simulink library "ServoCommand"  (R2014b)
settings: Solver=ode45  StartTime=0.0  StopTime=10.0  RelTol=1e-3
libraries: ServoCommand x12, simulink x6
settings Model: Creator=Sebastian  LastModifiedBy=Sebastian

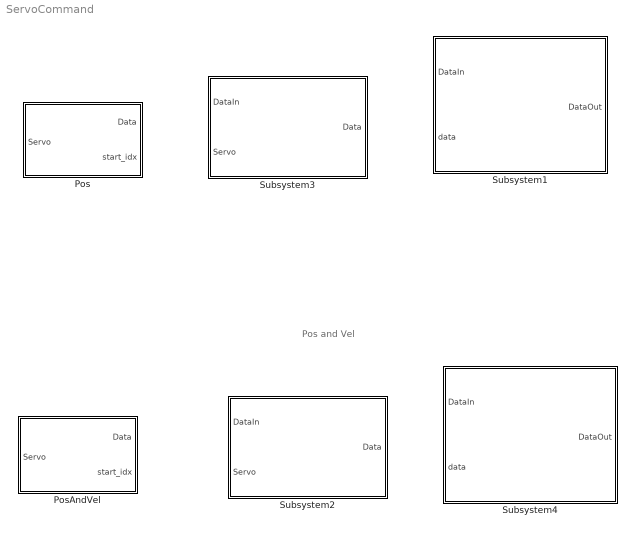
== system ServoCommand ==
  note: Pos and Vel
  Pos : Subsystem
  PosAndVel : Subsystem
  Subsystem1 : Subsystem
  Subsystem2 : Subsystem
  Subsystem3 : Subsystem
  Subsystem4 : Subsystem

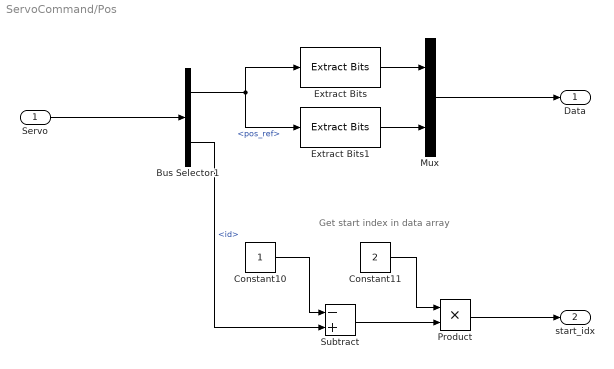
== system ServoCommand/Pos ==
  note: Get start index in data array
  Servo : Inport
  Bus Selector1 : BusSelector  OutputSignals=pos_ref,id
  Constant10 : Constant  OutDataTypeStr=uint8  SampleTime=-1
  Constant11 : Constant  Value=2  OutDataTypeStr=uint8  SampleTime=-1
  Extract Bits : simulink/Logic and Bit Operations/Extract Bits  bitsToExtract=Lower half  numBits=8  bitIdxRange=[0 7]  outScalingMode=Treat bit field as an integer
  Extract Bits1 : simulink/Logic and Bit Operations/Extract Bits  bitsToExtract=Upper half  numBits=8  bitIdxRange=[0 7]  outScalingMode=Treat bit field as an integer
  Mux : Mux  Inputs=2
  Product : Product
  Subtract : Sum  Inputs=-+
  Data : Outport
  start_idx : Outport  Port=2
  wires:
  Extract Bits/1 -> Mux/1
  Extract Bits1/1 -> Mux/2
  Servo/1 -> Bus Selector1/1
  Bus Selector1/1 -> Extract Bits/1, Extract Bits1/1  "<pos_ref>"
  Constant10/1 -> Subtract/1
  Subtract/1 -> Product/2
  Product/1 -> start_idx/1
  Constant11/1 -> Product/1
  Bus Selector1/2 -> Subtract/2  "<id>"
  Mux/1 -> Data/1

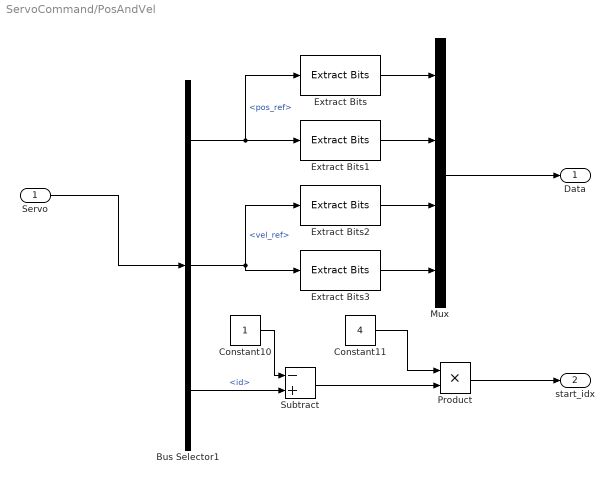
== system ServoCommand/PosAndVel ==
  Servo : Inport  OutDataTypeStr=Bus: Servo
  Bus Selector1 : BusSelector  OutputSignals=pos_ref,vel_ref,id
  Constant10 : Constant  OutDataTypeStr=uint8  SampleTime=-1
  Constant11 : Constant  Value=4  OutDataTypeStr=uint8  SampleTime=-1
  Extract Bits : simulink/Logic and Bit Operations/Extract Bits  bitsToExtract=Lower half  numBits=8  bitIdxRange=[0 7]  outScalingMode=Treat bit field as an integer
  Extract Bits1 : simulink/Logic and Bit Operations/Extract Bits  bitsToExtract=Upper half  numBits=8  bitIdxRange=[0 7]  outScalingMode=Treat bit field as an integer
  Extract Bits2 : simulink/Logic and Bit Operations/Extract Bits  bitsToExtract=Lower half  numBits=8  bitIdxRange=[0 7]  outScalingMode=Treat bit field as an integer
  Extract Bits3 : simulink/Logic and Bit Operations/Extract Bits  bitsToExtract=Upper half  numBits=8  bitIdxRange=[0 7]  outScalingMode=Treat bit field as an integer
  Mux : Mux
  Product : Product
  Subtract : Sum  Inputs=-+
  Data : Outport
  start_idx : Outport  Port=2
  wires:
  Extract Bits/1 -> Mux/1
  Extract Bits1/1 -> Mux/2
  Servo/1 -> Bus Selector1/1
  Bus Selector1/1 -> Extract Bits/1, Extract Bits1/1  "<pos_ref>"
  Constant10/1 -> Subtract/1
  Subtract/1 -> Product/2
  Product/1 -> start_idx/1
  Constant11/1 -> Product/1
  Bus Selector1/3 -> Subtract/2  "<id>"
  Mux/1 -> Data/1
  Extract Bits2/1 -> Mux/3
  Extract Bits3/1 -> Mux/4
  Bus Selector1/2 -> Extract Bits2/1, Extract Bits3/1  "<vel_ref>"

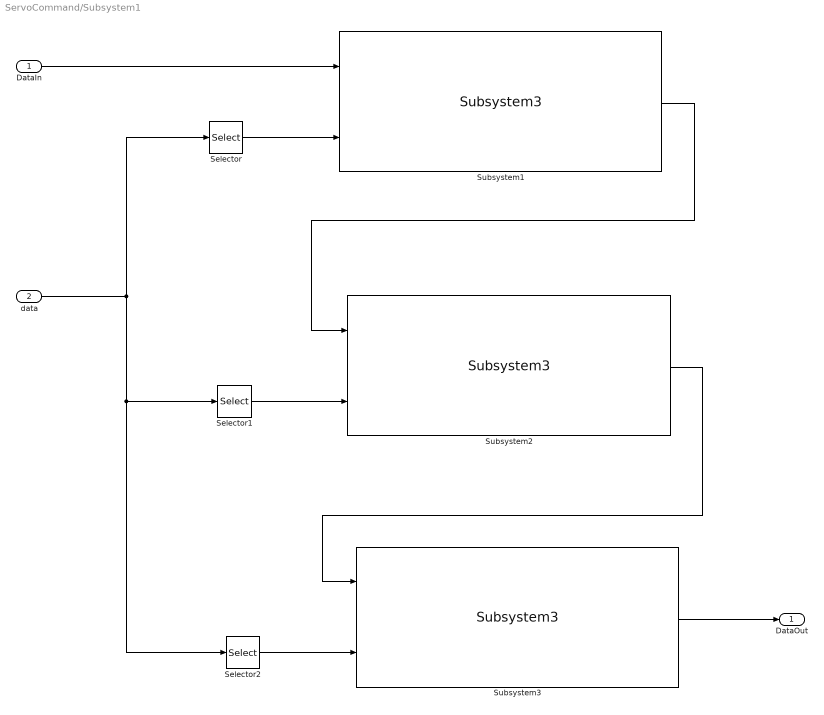
== system ServoCommand/Subsystem1 ==
  DataIn : Inport
  data : Inport  Port=2
  Selector : Selector  IndexMode=Zero-based  InputPortWidth=3  Indices=0
  Selector1 : Selector  IndexMode=Zero-based  InputPortWidth=3
  Selector2 : Selector  IndexMode=Zero-based  InputPortWidth=3  Indices=2
  Subsystem1 : ServoCommand/Subsystem3
  Subsystem2 : ServoCommand/Subsystem3
  Subsystem3 : ServoCommand/Subsystem3
  DataOut : Outport
  wires:
  Selector1/1 -> Subsystem2/2
  Subsystem2/1 -> Subsystem3/1
  data/1 -> Selector1/1, Selector2/1, Selector/1
  Selector2/1 -> Subsystem3/2
  Subsystem1/1 -> Subsystem2/1
  DataIn/1 -> Subsystem1/1
  Selector/1 -> Subsystem1/2
  Subsystem3/1 -> DataOut/1

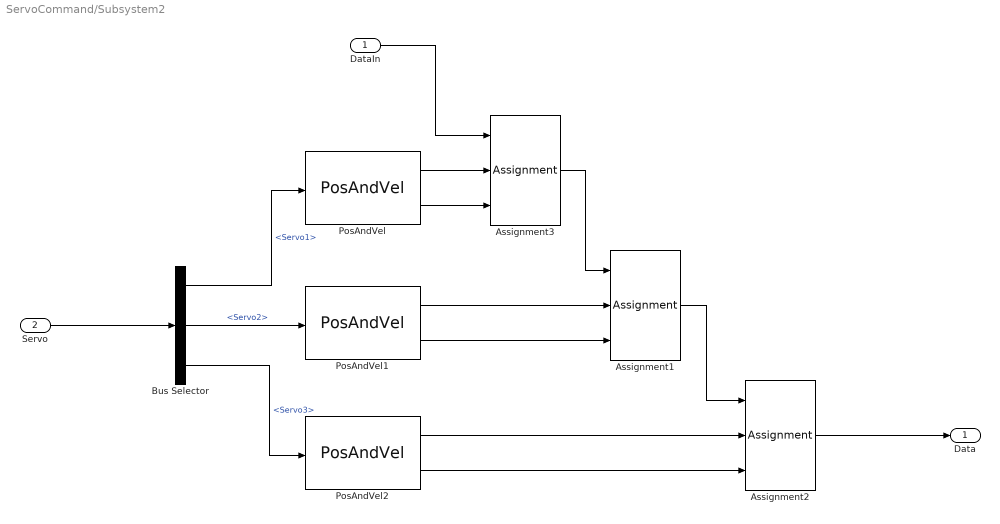
== system ServoCommand/Subsystem2 ==
  DataIn : Inport
  Servo : Inport  Port=2  OutDataTypeStr=Bus: Leg_ref
  Assignment1 : Assignment  IndexMode=Zero-based  IndexOptions=Starting index (port)  OutputSizes=36
  Assignment2 : Assignment  IndexMode=Zero-based  IndexOptions=Starting index (port)  OutputSizes=36
  Assignment3 : Assignment  IndexMode=Zero-based  IndexOptions=Starting index (port)  OutputSizes=36
  Bus Selector : BusSelector  OutputSignals=Servo1,Servo2,Servo3
  PosAndVel : ServoCommand/PosAndVel
  PosAndVel1 : ServoCommand/PosAndVel
  PosAndVel2 : ServoCommand/PosAndVel
  Data : Outport
  wires:
  Servo/1 -> Bus Selector/1
  Assignment2/1 -> Data/1
  DataIn/1 -> Assignment3/1
  PosAndVel2/2 -> Assignment2/3
  PosAndVel/1 -> Assignment3/2
  Bus Selector/3 -> PosAndVel2/1  "<Servo3>"
  PosAndVel/2 -> Assignment3/3
  PosAndVel1/1 -> Assignment1/2
  PosAndVel1/2 -> Assignment1/3
  Assignment1/1 -> Assignment2/1
  PosAndVel2/1 -> Assignment2/2
  Assignment3/1 -> Assignment1/1
  Bus Selector/2 -> PosAndVel1/1  "<Servo2>"
  Bus Selector/1 -> PosAndVel/1  "<Servo1>"

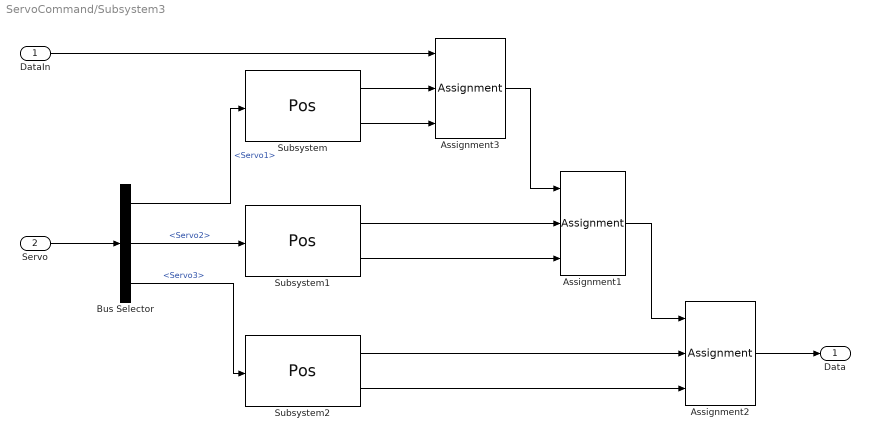
== system ServoCommand/Subsystem3 ==
  DataIn : Inport
  Servo : Inport  Port=2  OutDataTypeStr=Bus: Leg_ref
  Assignment1 : Assignment  IndexMode=Zero-based  IndexOptions=Starting index (port)  OutputSizes=36
  Assignment2 : Assignment  IndexMode=Zero-based  IndexOptions=Starting index (port)  OutputSizes=36
  Assignment3 : Assignment  IndexMode=Zero-based  IndexOptions=Starting index (port)  OutputSizes=36
  Bus Selector : BusSelector  OutputSignals=Servo1,Servo2,Servo3
  Subsystem : ServoCommand/Pos
  Subsystem1 : ServoCommand/Pos
  Subsystem2 : ServoCommand/Pos
  Data : Outport
  wires:
  Servo/1 -> Bus Selector/1
  Assignment2/1 -> Data/1
  Subsystem2/2 -> Assignment2/3
  Subsystem/1 -> Assignment3/2
  Bus Selector/3 -> Subsystem2/1  "<Servo3>"
  Subsystem/2 -> Assignment3/3
  Subsystem1/1 -> Assignment1/2
  Subsystem1/2 -> Assignment1/3
  Assignment1/1 -> Assignment2/1
  Subsystem2/1 -> Assignment2/2
  Assignment3/1 -> Assignment1/1
  Bus Selector/2 -> Subsystem1/1  "<Servo2>"
  Bus Selector/1 -> Subsystem/1  "<Servo1>"
  DataIn/1 -> Assignment3/1

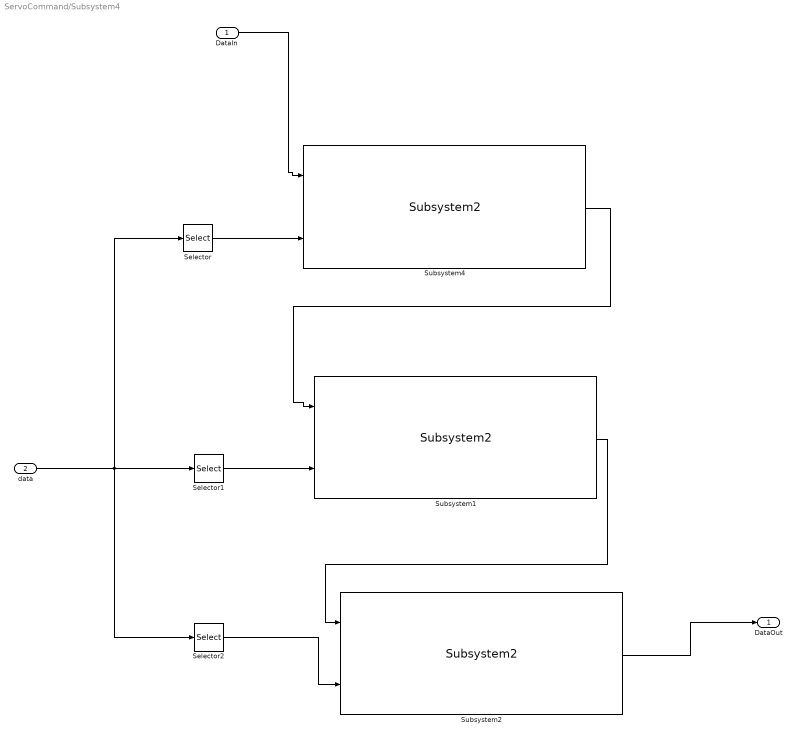
== system ServoCommand/Subsystem4 ==
  DataIn : Inport
  data : Inport  Port=2
  Selector : Selector  IndexMode=Zero-based  InputPortWidth=3  Indices=0
  Selector1 : Selector  IndexMode=Zero-based  InputPortWidth=3
  Selector2 : Selector  IndexMode=Zero-based  InputPortWidth=3  Indices=2
  Subsystem1 : ServoCommand/Subsystem2
  Subsystem2 : ServoCommand/Subsystem2
  Subsystem4 : ServoCommand/Subsystem2
  DataOut : Outport
  wires:
  Selector1/1 -> Subsystem1/2
  Subsystem1/1 -> Subsystem2/1
  data/1 -> Selector/1, Selector1/1, Selector2/1
  Selector2/1 -> Subsystem2/2
  Subsystem4/1 -> Subsystem1/1
  DataIn/1 -> Subsystem4/1
  Selector/1 -> Subsystem4/2
  Subsystem2/1 -> DataOut/1
